simulink model "Controlled_DoubleTank_simul"  (R2018b)
settings: Solver=VariableStepAuto  StartTime=0.0  StopTime=200  FixedStep=0.001  RelTol=1e-3
values from neighbouring files (symbols this model uses):
  A = [0.967743748526  0; 0.031730333008  0.967743748526]    [Dados_Tanques.mat]    (also in double_tank_simu.m = sysd.A; nma_simplex.m = tab(1:nRow-1,1:nCol-1); nma_simplex_2.m = tab(1:nRow-1,1:nCol-1))
  a1 = 0.17795237427    [Dados_Tanques.mat]    (also in double_tank_simu.m)
  A1 = 15.5179165474    [Dados_Tanques.mat]    (also in double_tank_simu.m)
  A2 = 15.5179165474    [Dados_Tanques.mat]    (also in double_tank_simu.m)
  a2 = 0.17795237427    [Dados_Tanques.mat]    (also in double_tank_simu.m)
  B = [0.104604453049 0.0017055116738]    [Dados_Tanques.mat]    (also in double_tank_simu.m = sysd.B)
  g = 981    [Dados_Tanques.mat]    (also in double_tank_simu.m)
  Gv = [1 -1 0 0 0.0316763086938 -0.0316763086938 0.0610064360648 -0.0610064360648 0.0878578258116 -0.0878578258116 0.112163466595 -0.112163466595 ... (32 elements, 16x2)]    [Dados_Tanques.mat]
  km = 3.3    [Dados_Tanques.mat]    (also in double_tank_simu.m = 4.1)
  ncu = 1    [Dados_Tanques.mat]
  nlu = 2    [Dados_Tanques.mat]
  phi = [2.74907887757 9.25092112243]    [Dados_Tanques.mat]    (also in double_tank_simu.m = [(12-ueq) ueq]')
  rhov = [15 15 15 15 14.8404669643 14.8293968766 14.6652011254 14.6221983313 14.4769073428 14.3832726141 14.2782768412 14.1176408708 ... (16 elements, 16x1)]    [Dados_Tanques.mat]
  U = [1 -1]    [Dados_Tanques.mat]    (also in double_tank_simu.m = [1 -1]')
  ueq = 9.25092112243    [Dados_Tanques.mat]    (also in double_tank_simu.m = (a1/km)*sqrt(2*g*x1eq))
  x1eq = 15    [Dados_Tanques.mat]    (also in double_tank_simu.m = (1/(2*g))*((km*ueq)/a1)^2)
  x2eq = 15    [Dados_Tanques.mat]    (also in double_tank_simu.m)
undefined symbols (not defined in the file or in its folder): control
settings Model: Creator=Tiago Alves  LastModifiedBy=Tiago Alves

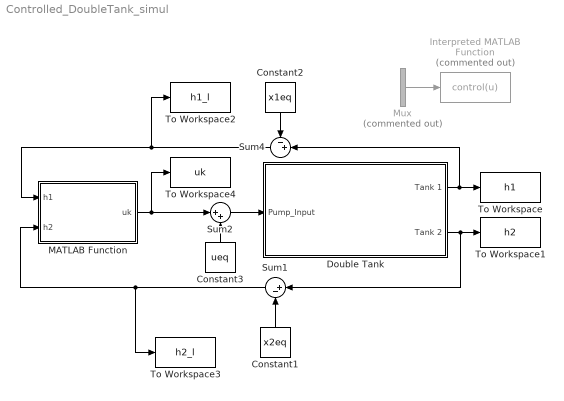
== system Controlled_DoubleTank_simul ==
  Constant1 : Constant  Value=x2eq
  Constant2 : Constant  Value=x1eq
  Constant3 : Constant  Value=ueq
  Double Tank : Subsystem
  Interpreted MATLAB Function : MATLABFcn  Commented=on  MATLABFcn=control(u)
  MATLAB Function : MATLAB Function  TreatAsAtomicUnit=on
  Mux : Mux  Commented=on  Inputs=2
  Sum1 : Sum  Inputs=|+-
  Sum2 : Sum  Inputs=|++
  Sum4 : Sum  Inputs=-+|
  To Workspace : ToWorkspace  VariableName=h1  SaveFormat=Timeseries  SampleTime=-1
  To Workspace1 : ToWorkspace  VariableName=h2  SaveFormat=Timeseries  SampleTime=-1
  To Workspace2 : ToWorkspace  VariableName=h1_l  SaveFormat=Timeseries  SampleTime=-1
  To Workspace3 : ToWorkspace  VariableName=h2_l  SaveFormat=Timeseries  SampleTime=-1
  To Workspace4 : ToWorkspace  VariableName=uk  SaveFormat=Timeseries  SampleTime=-1
  wires:
  Double Tank/1(Tank 1) -> Sum4/2, To Workspace/1
  Double Tank/2(Tank 2) -> To Workspace1/1, Sum1/1
  Sum4/1 -> MATLAB Function/1(h1), To Workspace2/1
  Constant2/1 -> Sum4/1
  Constant1/1 -> Sum1/2
  Sum1/1 -> MATLAB Function/2(h2), To Workspace3/1
  Constant3/1 -> Sum2/2
  Sum2/1 -> Double Tank/1(Pump_Input)
  MATLAB Function/1(uk) -> To Workspace4/1, Sum2/1
  Mux/1 -> Interpreted MATLAB Function/1

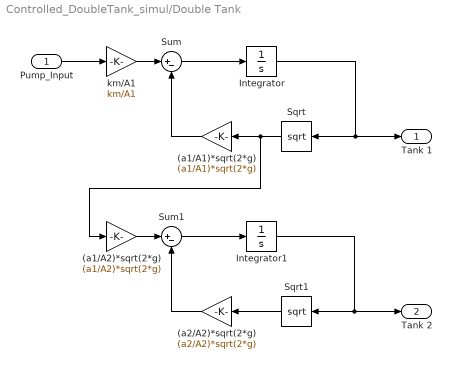
== system Controlled_DoubleTank_simul/Double Tank ==
  Pump_Input : Inport
  (a1/A1)*sqrt(2*g) : Gain  Gain=(a1/A1)*sqrt(2*g)
  (a1/A2)*sqrt(2*g) : Gain  Gain=(a1/A2)*sqrt(2*g)
  (a2/A2)*sqrt(2*g) : Gain  Gain=(a2/A2)*sqrt(2*g)
  Integrator : Integrator  InitialCondition=15+5
  Integrator1 : Integrator  InitialCondition=15+5
  Sqrt : Sqrt  SaturateOnIntegerOverflow=on
  Sqrt1 : Sqrt  SaturateOnIntegerOverflow=on
  Sum : Sum  Inputs=|+-
  Sum1 : Sum  Inputs=|+-
  km/A1 : Gain  Gain=km/A1
  Tank 1 : Outport
  Tank 2 : Outport  Port=2
  wires:
  km/A1/1 -> Sum/1
  Integrator/1 -> Sqrt/1, Tank 1/1
  (a1/A2)*sqrt(2*g)/1 -> Sum1/1
  Sqrt/1 -> (a1/A2)*sqrt(2*g)/1, (a1/A1)*sqrt(2*g)/1
  Sum/1 -> Integrator/1
  (a2/A2)*sqrt(2*g)/1 -> Sum1/2
  Sum1/1 -> Integrator1/1
  (a1/A1)*sqrt(2*g)/1 -> Sum/2
  Sqrt1/1 -> (a2/A2)*sqrt(2*g)/1
  Pump_Input/1 -> km/A1/1
  Integrator1/1 -> Tank 2/1, Sqrt1/1

== matlab function Controlled_DoubleTank_simul/MATLAB Function ==
  data: h1 input; uk output; h2 input; ncu parameter; Gv parameter; B parameter; rhov parameter; U parameter; nlu parameter; A parameter; phi parameter
%%%%%%%%%%%%%%%%%%%%%%%%%%%%%%%%%%%%
% STATIC STATE FEEDBACK CONTROLLER %
%%%%%%%%%%%%%%%%%%%%%%%%%%%%%%%%%%%%

function uk = fcn(h1, h2, ncu, Gv, B, rhov, U, nlu, A, phi)
    
    %coder.extrinsic('nma_simplex');
    xk = [h1 h2]';
    %fobj = [zeros(ncu, 1); 1];
    fobj = [zeros(ncu, 1) 1 zeros(1,18)]; 
    %Apo = [Gv*B -rhov; U zeros(nlu, 1)];
    Apo = [[Gv*B -rhov; U zeros(nlu, 1)] eye(18)];
    Bpo = [-Gv*A*xk; phi];
    
    %       arg    min     epsi
    %            u,epsi
    %
    %         |Gv*B  -rhov|       | -Gv*A*xk |
    % Apo   = |  U     0  | Bpo = |    phi   |

    %v = linprog(fobj, Apo, Bpo);
    sol = nma_simplex(Apo,Bpo,fobj,false);
    %uk = v(1);
    %epsi_LP = [epsi_LP v(2)];

uk = sol(1);
end
function sol = nma_simplex(Aa,b,c,debug)
%function [A,b,c]=nma_simplex(A,b,c)
%This function implments the simplex matrix algorithm.
%It accepts A_eq and b_eq and c as defined in standard 
%documentation and generates all the simplex tableaus, and 
%returns the final tableau which the user can read from it the 
%minimum value of the objective function and the optimal x vector 
%directly.
%
%It runs both phase one and phase two automatically.
%
%The input is
%
%A: This is the Ax=b matrix. This is for simplex standard 
%   form only. The caller must convert all inequalites to 
%   equalities first by using slack and suprluse variables. This 
%   is what is called the Aeq matrix in Matlab documenation. 
%   This function does not support Ax<b form. A has to be in 
%   standard form
%
%b: Vector. This is the right hand side of Ax=b.
%
%c: Vector. This is from minimize  J(x) = c'x. As defined in 
%   standard Matlab documentations.
%
%debug: flag. Set to true to see lots of internal steps.
%
%Returns:
%
%This function returns the final tableau. It has the form
%
%  [ A | b  ]
%  [ c | J  ]
%
% UPDATES
%
% Version May 12,  2016   original
% Version June 17, 2020   updated to print the final solution vector
%                         to make it easier to read.
% by Nasser M. Abbasi
% Free for use.

validate_input(Aa,b,c);

[Aa,b] = make_phase_one(Aa,b,debug);
tab   = simplex(Aa,b,c,debug,'phase two')
sol = print_solution_vector(tab);
end
%==========================
function [Aa,b] = make_phase_one(Aa,b,debug)
[m,n]              = size(Aa);
tab                = zeros(m+1,n+m+1);
tab(1:m,1:n)       = Aa;
tab(end,n+1:end-1) = 1;
tab(1:m,end)       = b(:);
tab(1:m,n+1:n+m)   = eye(m);

if debug
    fprintf('>>>>Current tableau [phase one]\n');
    disp(tab);
end

for i = 1:m %now make all entries in bottom row zero
    tab(end,:) = tab(end,:)-tab(i,:);
end

tab = simplex(tab(1:m,1:n+m),tab(1:m,end),tab(end,1:n+m),...
                                             debug,'phase one');
%if tab(end,end) ~=0
%   error('artificial J(x) is not zero at end of phase one.');
%end

Aa = tab(1:m,1:n);
b = tab(1:m,end);

end
%=================================
function tab = simplex(Aa,b,c,debug,phase_name)
[m,n]        = size(Aa);
tab          = zeros(m+1,n+1);
tab(1:m,1:n) = Aa;
tab(m+1,1:n) = c(:);
tab(1:m,end) = b(:);

keep_running = true;
while keep_running
    if debug
        fprintf('***********************\n');
        fprintf('Current tableau [%s] \n',phase_name);
        disp(tab);
    end
    
    if any(tab(end,1:n)<0)%check if there is negative cost coeff.
        [~,J] = min(tab(end,1:n)); %yes, find the most negative
        % now check if corresponding column is unbounded
        if all(tab(1:m,J)<=0) 
          error('problem unbounded. All entries <= 0 in column %d',J);
        %do row operations to make all entries in the column 0 
        %except pivot
        else 
            pivot_row = 0;
            min_found = inf;
            for i = 1:m
                if tab(i,J)>0
                    tmp = tab(i,end)/tab(i,J);
                    if tmp < min_found
                        min_found = tmp;
                        pivot_row = i;
                    end
                end
            end
            if debug
                fprintf('pivot row is %d\n',pivot_row);
            end
            %normalize
            tab(pivot_row,:) = tab(pivot_row,:)/tab(pivot_row,J); 
            %now make all entries in J column zero.
            for i=1:m+1
                if i ~= pivot_row
                    tab(i,:)=tab(i,:)-sign(tab(i,J))*...
                                 abs(tab(i,J))*tab(pivot_row,:);
                end
            end
        end
        if debug  %print current basic feasible solution
            fprintf('current basic feasible solution is\n');
            disp(get_current_x());
        end
    else
        keep_running=false;       
    end
end

    %internal function, finds current basis vector
    function current_x = get_current_x()
        current_x = zeros(n,1);
        for j=1:n
            if length(find(tab(:,j)==0))==m
                idx= tab(:,j)==1;
                current_x(j)=tab(idx,end);
            end
        end
    end
end
%==========================
function validate_input(Aa,b,c)
if ~ismatrix(Aa)
    error('A must be matrix');
end

if ~isvector(b)
    error('b must be vector');
end
if ~isvector(c)
    error('c must be vector');
end

[m,n]=size(Aa);
if rank(Aa) <m
    error('Rank A must be equal to number of rows in A');
end

if length(b) ~= m
    error('b must have same size as number of rows of A');
end
if length(c) ~= n
    error('c must have same size as number of columns of A');
end
end

%=================================
function solution_vector = print_solution_vector(tab)
%tab(1:m,1:n) = A;

[nRow,nCol] = size(tab);

A = tab(1:nRow-1,1:nCol-1);
b = tab(1:nRow-1,nCol);

q = A ~= 0;
q = find(sum(q,1)==1); %find all columns with one non-zero entry;

solution_vector = zeros(nCol-1,1); 

for n=1:length(q)
    j = find(A(1:nRow-1,q(n))==1);
    if isempty(j)
       solution_vector(q(n)) = 0;
    else
       solution_vector(q(n)) = b(j); 
    end
end

end
